simulink model "Modelo"  (R2016a)
settings: Solver=VariableStepAuto  StartTime=0.0  StopTime=30.0  RelTol=1e-3
values from neighbouring files (symbols this model uses):
  C = ss1.C    [MVE.m]
  G = ss1.A    [MVE.m]
  H = ss1.B    [MVE.m]
  K1 = Ktemp(1)    [MVE.m]
  K2 = Ktemp(2:end)    [MVE.m]
  Ke = acker(G',C',P)'    [MVE.m]
  Ts = 0.1    [MVE.m]
settings Model: Creator=Erick Eduarte  LastModifiedBy=luisd

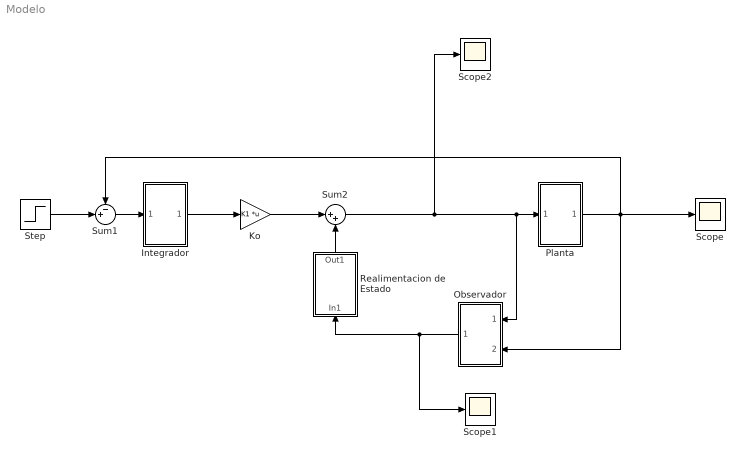
== system Modelo ==
  Integrador : Subsystem
  Ko : Gain  Gain=K1  Multiplication=Matrix(K*u)
  Observador : Subsystem
  Planta : Subsystem
  Realimentacion de Estado : Subsystem
  Scope : Scope
  Scope1 : Scope
  Scope2 : Scope
  Step : Step  After=2  SampleTime=Ts
  Sum1 : Sum  Inputs=-+|
  Sum2 : Sum  Inputs=|++
  wires:
  Sum2/1 -> Scope2/1, Observador/1(In1), Planta/1(In1)
  Ko/1 -> Sum2/1
  Realimentacion de Estado/1(Out1) -> Sum2/2
  Observador/1(Out1) -> Scope1/1, Realimentacion de Estado/1(In1)
  Integrador/1(Out1) -> Ko/1
  Sum1/1 -> Integrador/1(In1)
  Step/1 -> Sum1/2
  Planta/1(Out1) -> Sum1/1, Observador/2(In2), Scope/1

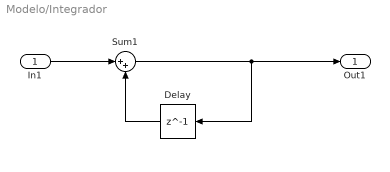
== system Modelo/Integrador ==
  In1 : Inport
  Delay : Delay  DelayLength=1  InitialCondition=0
  Sum1 : Sum  Inputs=|++
  Out1 : Outport
  wires:
  Sum1/1 -> Out1/1, Delay/1
  In1/1 -> Sum1/1
  Delay/1 -> Sum1/2

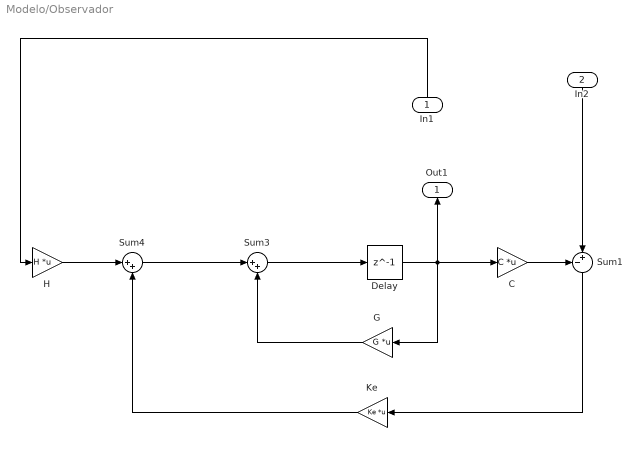
== system Modelo/Observador ==
  In1 : Inport
  In2 : Inport  Port=2
  C : Gain  Gain=C  Multiplication=Matrix(K*u)
  Delay : Delay  DelayLength=1  InitialCondition=1  SampleTime=0.1
  G : Gain  Gain=G  Multiplication=Matrix(K*u)
  H : Gain  Gain=H  Multiplication=Matrix(K*u)
  Ke : Gain  Gain=Ke  Multiplication=Matrix(K*u)
  Sum1 : Sum  Inputs=-+|
  Sum3 : Sum  Inputs=|++
  Sum4 : Sum  Inputs=|++
  Out1 : Outport
  wires:
  In2/1 -> Sum1/2
  Ke/1 -> Sum4/2
  G/1 -> Sum3/2
  C/1 -> Sum1/1
  Delay/1 -> Out1/1, G/1, C/1
  Sum4/1 -> Sum3/1
  In1/1 -> H/1
  Sum3/1 -> Delay/1
  H/1 -> Sum4/1
  Sum1/1 -> Ke/1

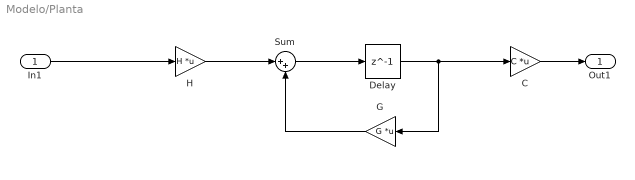
== system Modelo/Planta ==
  In1 : Inport
  C : Gain  Gain=C  Multiplication=Matrix(K*u)
  Delay : Delay  DelayLength=1  InitialCondition=1  SampleTime=0.1
  G : Gain  Gain=G  Multiplication=Matrix(K*u)
  H : Gain  Gain=H  Multiplication=Matrix(K*u)
  Sum : Sum  Inputs=|++
  Out1 : Outport
  wires:
  Delay/1 -> C/1, G/1
  C/1 -> Out1/1
  Sum/1 -> Delay/1
  G/1 -> Sum/2
  H/1 -> Sum/1
  In1/1 -> H/1

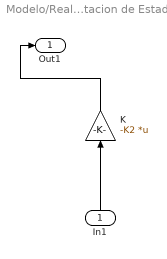
== system Modelo/Realimentacion de Estado ==
  In1 : Inport
  K : Gain  Gain=-K2  Multiplication=Matrix(K*u)
  Out1 : Outport
  wires:
  K/1 -> Out1/1
  In1/1 -> K/1
